simulink model "vlowpass"  (R2022a)
settings: Solver=ode4  StartTime=0.0  StopTime=inf  FixedStep=1/400  RelTol=1e-3
libraries: aerolibconvert2 x2, sharedtransform x2, eeGeneralControl x1
settings Model: Creator=kcx06  LastModifiedBy=kcx06

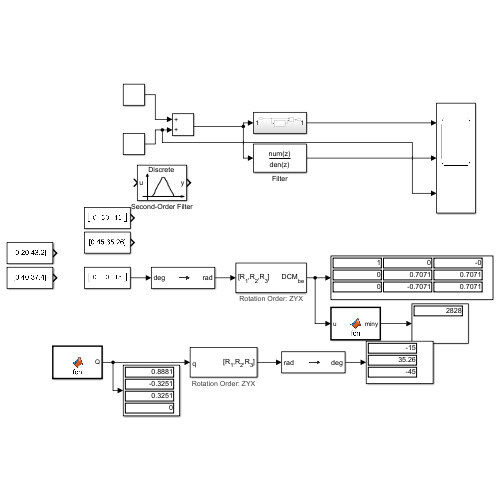
[thumbnail: Simulink's stored preview of the top-level diagram]
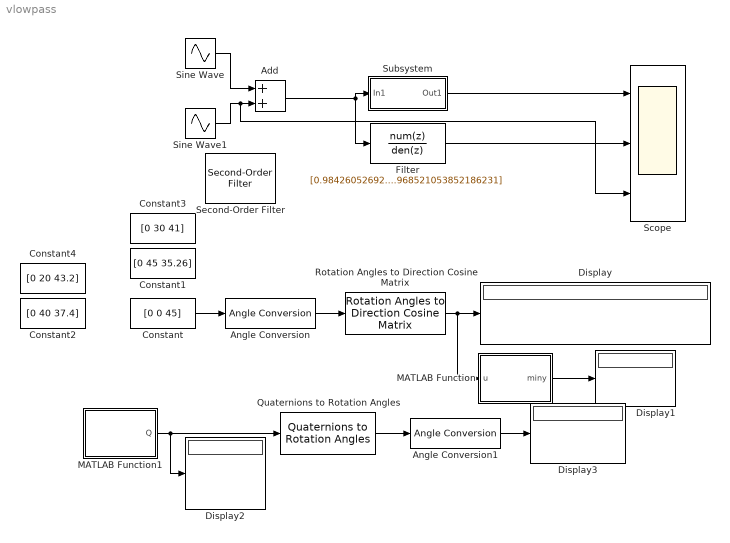
== system vlowpass ==
  Add : Sum
  Angle Conversion : aerolibconvert2/Angle Conversion  IU=deg  OU=rad
  Angle Conversion1 : aerolibconvert2/Angle Conversion  IU=rad  OU=deg
  Constant : Constant  Value=[0 0 45]
  Constant1 : Constant  Value=[0 45 35.26]
  Constant2 : Constant  Value=[0 40 37.4]
  Constant3 : Constant  Value=[0 30 41]
  Constant4 : Constant  Value=[0 20 43.2]
  Display{,1..3} (4 alike) : Display
  Filter : DiscreteFilter  Tag=BlockMethodSubSystem  Numerator=[0.984260526926093116 -1.90667634508841477 0.984260526926093116]  Denominator=[1 -1.90667634508841477 0.968521053852186231]  SampleTime=1/100  a0EqualsOne=on
  MATLAB Function : MATLAB Function  TreatAsAtomicUnit=on
  MATLAB Function1 : MATLAB Function  TreatAsAtomicUnit=on
  Quaternions to Rotation Angles : sharedtransform/Quaternions to Rotation Angles  rotationOrder=ZYX  aMode=aMode
      settings: SourceProductBaseCode=AE,PW,DR,MT,VE
  Rotation Angles to Direction Cosine Matrix : sharedtransform/Rotation Angles to Direction Cosine Matrix  rotationOrder=ZYX  aMode=aMode
      settings: SourceProductBaseCode=AE,PW,DR,MT,VE
  Scope : Scope  NumInputPorts=3
  Second-Order Filter : eeGeneralControl/Second-Order Filter  FilterType=Band-pass  fn=4  Zeta=0.707  Ts=1/100  A0=0  Ph0=0  f0=0  b0=0
      settings: SourceProductBaseCode=PS
  Sine Wave : Sin  Frequency=4*2*pi  SampleTime=1/100
  Sine Wave1 : Sin  Amplitude=5  Frequency=4*0.2*pi  SampleTime=1/100
  Subsystem : Subsystem
  wires:
  Sine Wave1/1 -> Scope/3, Add/2
  Sine Wave/1 -> Add/1
  Add/1 -> Filter/1, Subsystem/1(In1)
  Subsystem/1(Out1) -> Scope/1
  Filter/1 -> Scope/2
  Constant/1 -> Angle Conversion/1
  Rotation Angles to Direction Cosine Matrix/1 -> MATLAB Function/1(u), Display/1
  MATLAB Function/1(miny) -> Display1/1
  Angle Conversion/1 -> Rotation Angles to Direction Cosine Matrix/1
  MATLAB Function1/1(Q) -> Quaternions to Rotation Angles/1, Display2/1
  Quaternions to Rotation Angles/1 -> Angle Conversion1/1
  Angle Conversion1/1 -> Display3/1

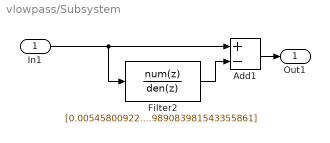
== system vlowpass/Subsystem ==
  In1 : Inport
  Add1 : Sum  Inputs=+-
  Filter2 : DiscreteFilter  Tag=BlockMethodSubSystem  Numerator=[0.00545800922832206936 0 -0.00545800922832206936]  Denominator=[1 -1.92659325059358721 0.989083981543355861]  a0EqualsOne=on
  Out1 : Outport
  wires:
  Filter2/1 -> Add1/2
  In1/1 -> Add1/1, Filter2/1
  Add1/1 -> Out1/1

== matlab function vlowpass/MATLAB Function ==
  data: u input; miny output
function miny = fcn(u)
y = abs([2000/u(3,1);
2000/u(3,2);
2000/u(3,3)]);
miny = min(y);

== matlab function vlowpass/MATLAB Function1 ==
  data: Q output
function Q = fcn()
angle = acos(1/sqrt(3));
Q =[cos(angle/2), -1/sqrt(2)*sin(angle/2),1/sqrt(2)*sin(angle/2),0*sin(angle/2)]
